simulink model "stablechange"  (R2024b)
settings: Solver=ode45  StartTime=0.0  StopTime=10  FixedStep=1e-5  MaxStep=1e-4  RelTol=1e-3
undefined symbols (not defined in the file): X, Y, Z
libraries: sm_lib x17, nesl_utility x17
settings Model: Creator=lxr  LastModifiedBy=lxr
settings DataIOCC: InspectSignalLogs=on
settings ExplorerConfigSet: InternalSimMechanicsExplorerSettings="<ExplorerConfiguration><canonicalview>default</canonicalview><AnimationSetting><BasePlaybackSpeed>1.0</BasePlaybackSpeed><PlaybackSpeedFactor>1.0</PlaybackSpeedFactor></AnimationSetting><TilePanel><TileInfo><Tiles Columns=\"1\" Count=\"1\" Rows=\"1\"><Column Weight=\"1\"/><Row Weight=\"1\"/><Tile Height=\"1\" Width=\"1\" X=\"0\" Y=\"0\"/></Tiles></TileInfo><SceneInfo><SceneViewer><BGColor><R>0.60000002384185791</R><G>0.60000002384185791</G><B>0.60000002384185791</B></BGColor><Camera><DoPerspective>off</DoPerspective><Position><X>0.439437272864546535</X><Y>-2.25247873719255853</Y><Z>0.67311615033412453</Z></Position><Center><X>0.439437272864546535</X><Y>-2.22044604925031308e-16</Y><Z>0.67311615033412453</Z></Center><Up><X>0</X><Y>-0</Y><Z>1</Z></Up><ViewLimDist>1</ViewLimDist><YLim>3.10627937128803433</YLim><XLim>4.75624821439115486</XLim></Camera></SceneViewer></SceneInfo></TilePanel><MechEditorPanel><Cameras/><GfxPanelCameraMap/><VideoCreator><PlaybackSpeedRatio>1.0</PlaybackSpeedRatio><FrameRate>30</FrameRate><VideoFormat>Motion JPEG AVI</VideoFormat><FrameSize>auto</FrameSize></VideoCreator></MechEditorPanel></ExplorerConfiguration>"

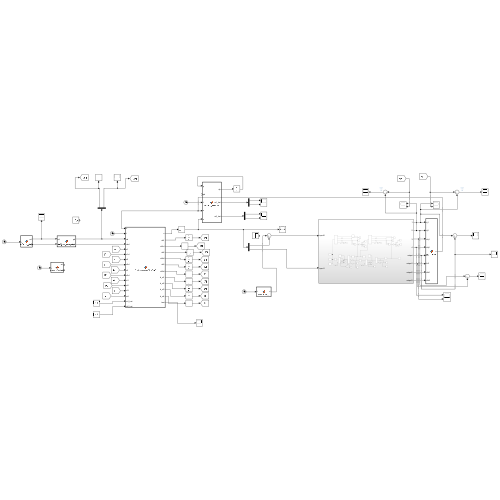
[thumbnail: Simulink's stored preview of the top-level diagram]
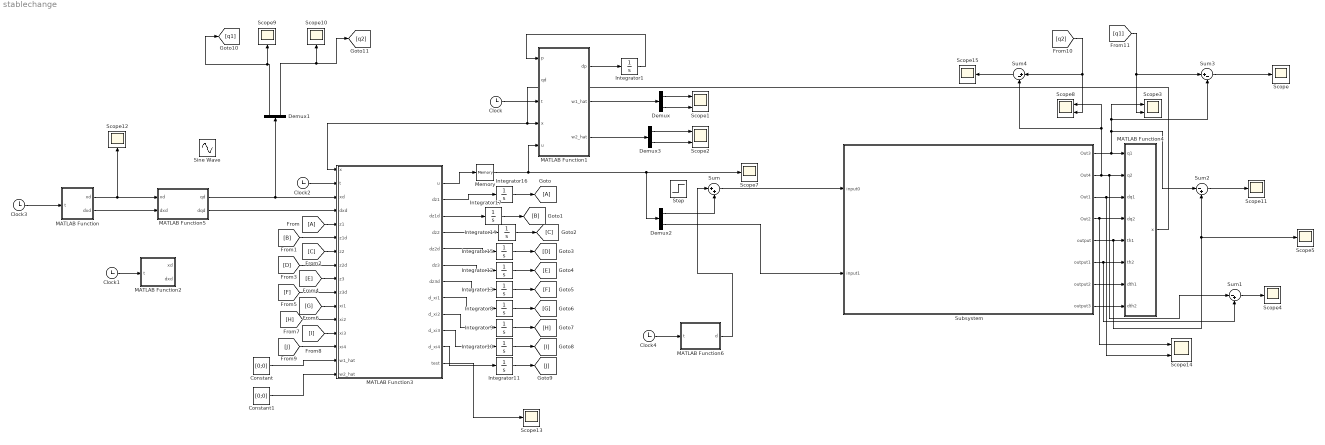
== system stablechange ==
  Clock{,1..4} (5 alike) : Clock
  Constant : Constant  Value=[0;0]
  Constant1 : Constant  Value=[0;0]
  Demux{,1..3} (4 alike) : Demux  Outputs=2
  From : From
  Goto : Goto
  Integrator1 : Integrator  InitialCondition=[0; 0; 0; 0]
  Integrator{8..11,13..17} (9 alike) : Integrator  InitialCondition=[0; 0]
  Integrator12 : Integrator  InitialCondition=[18.5625;135.5175]
  MATLAB Function : MATLAB Function  TreatAsAtomicUnit=on
  MATLAB Function1 : MATLAB Function  TreatAsAtomicUnit=on
  MATLAB Function2 : MATLAB Function  TreatAsAtomicUnit=on
  MATLAB Function3 : MATLAB Function  TreatAsAtomicUnit=on
  MATLAB Function4 : MATLAB Function  TreatAsAtomicUnit=on
  MATLAB Function5 : MATLAB Function  TreatAsAtomicUnit=on
  MATLAB Function6 : MATLAB Function  TreatAsAtomicUnit=on
  Memory : Memory
  Scope{,4..5,7,9..13,15} (10 alike) : Scope
  Scope{1..3,8,14} (5 alike) : Scope  NumInputPorts=2
  Sine Wave : Sin  Amplitude=5  Frequency=100  SampleTime=0
  Step : Step  Time=0  After=5  SampleTime=0
  Subsystem : Subsystem
  Sum : Sum  Inputs=|++
  Sum1 : Sum  Inputs=|-+
  Sum2 : Sum  Inputs=|-+
  Sum3 : Sum  Inputs=|+-
  Sum4 : Sum  Inputs=|+-
  wires:
  MATLAB Function3/11(d_xi4) -> Integrator11/1
  Sum2/1 -> Scope11/1
  MATLAB Function3/9(d_xi2) -> Integrator9/1
  Subsystem/3(Out1) -> Scope14/2, MATLAB Function4/3(dq1)
  [B] -> MATLAB Function3/6(z1d)
  Integrator9/1 -> [H]
  MATLAB Function3/10(d_xi3) -> Integrator10/1
  [J] -> MATLAB Function3/14(xi4)
  Integrator1/1 -> MATLAB Function1/1(p)
  MATLAB Function3/4(dz2) -> Integrator14/1
  Demux1/1 -> [q1], Scope9/1
  Subsystem/8(output3) -> MATLAB Function4/8(dth2)
  Demux2/2 -> Subsystem/2(input1)
  Subsystem/1(Out3) -> Sum2/1, Sum3/2, Scope3/1, MATLAB Function4/1(q1)
  Integrator13/1 -> [F]
  MATLAB Function3/5(dz2d) -> Integrator15/1
  Subsystem/7(output2) -> MATLAB Function4/7(dth1)
  MATLAB Function4/1(x) -> MATLAB Function3/1(x), MATLAB Function1/4(x)
  Integrator15/1 -> [D]
  MATLAB Function3/6(dz3) -> Integrator12/1
  Subsystem/5(output) -> Scope5/1, Sum2/2, MATLAB Function4/5(th1)
  Subsystem/2(Out4) -> Sum4/2, Scope8/1, Sum1/1, MATLAB Function4/2(q2)
  [C] -> MATLAB Function3/7(z2)
  Demux1/2 -> [q2], Scope10/1
  MATLAB Function3/3(dz1d) -> Integrator17/1
  [E] -> MATLAB Function3/9(z3)
  Integrator8/1 -> [G]
  Subsystem/6(output1) -> Sum1/2, MATLAB Function4/6(th2)
  Subsystem/4(Out2) -> Scope14/1, MATLAB Function4/4(dq2)
  From/1 -> MATLAB Function3/5(z1)
  Integrator16/1 -> Goto/1
  MATLAB Function1/1(dp) -> Integrator1/1
  MATLAB Function3/7(dz3d) -> Integrator13/1
  [I] -> MATLAB Function3/13(xi3)
  Integrator10/1 -> [I]
  [H] -> MATLAB Function3/12(xi2)
  Integrator17/1 -> [B]
  MATLAB Function3/2(dz1) -> Integrator16/1
  Integrator11/1 -> [J]
  MATLAB Function3/1(u) -> Memory/1
  Integrator12/1 -> [E]
  MATLAB Function3/8(d_xi1) -> Integrator8/1
  [D] -> MATLAB Function3/8(z2d)
  Integrator14/1 -> [C]
  [G] -> MATLAB Function3/11(xi1)
  [F] -> MATLAB Function3/10(z3d)
  Memory/1 -> MATLAB Function1/5(u), Scope7/1, Demux2/1
  Clock/1 -> MATLAB Function1/3(t)
  MATLAB Function1/2(w1_hat) -> Demux/1
  MATLAB Function1/3(w2_hat) -> Demux3/1
  Clock2/1 -> MATLAB Function3/2(t)
  Demux2/1 -> Sum/2
  Sum/1 -> Subsystem/1(input0)
  [q1] -> Sum3/1, Scope3/2
  [q2] -> Sum4/1, Scope8/2
  Sum1/1 -> Scope4/1
  Clock3/1 -> MATLAB Function/1(t)
  MATLAB Function/1(xd) -> Scope12/1, MATLAB Function5/1(xd)
  MATLAB Function/2(dxd) -> MATLAB Function5/2(dxd)
  MATLAB Function3/12(test) -> Scope13/1
  Sum4/1 -> Scope15/1
  Clock1/1 -> MATLAB Function2/1(t)
  Sum3/1 -> Scope/1
  Clock4/1 -> MATLAB Function6/1(t)
  Demux/1 -> Scope1/1
  Demux/2 -> Scope1/2
  Demux3/1 -> Scope2/1
  Demux3/2 -> Scope2/2
  MATLAB Function5/1(qd) -> Demux1/1, MATLAB Function3/3(xd)
  MATLAB Function5/2(dqd) -> MATLAB Function3/4(dxd)
  MATLAB Function6/1(d) -> Sum/1
  Constant/1 -> MATLAB Function3/15(w1_hat)
  Constant1/1 -> MATLAB Function3/16(w2_hat)

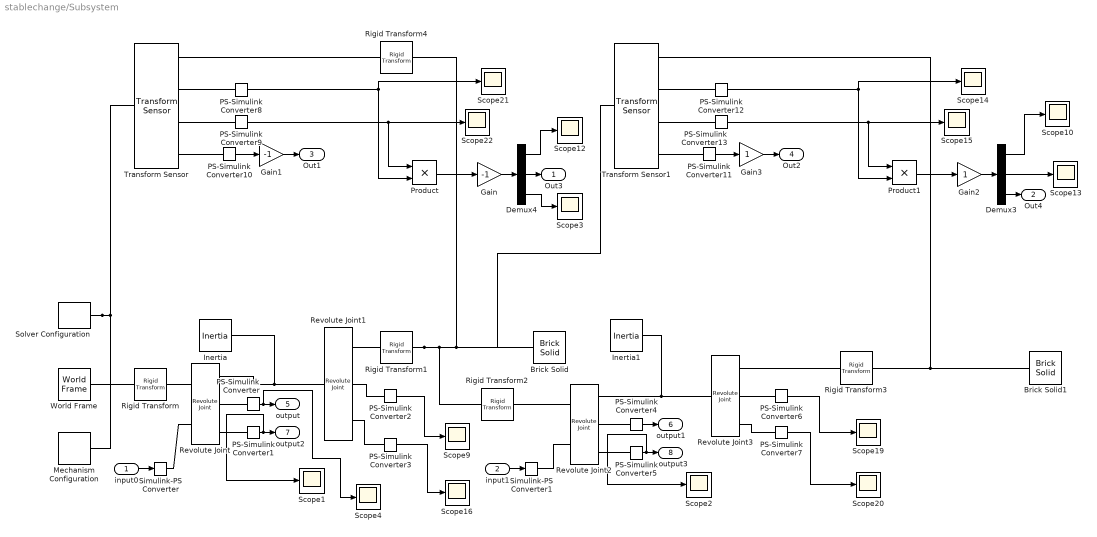
== system stablechange/Subsystem ==
  input0 : Inport
  input1 : Inport  Port=2
  Brick Solid : sm_lib/Body Elements/Brick Solid  BrickDimensions=[0.1 1.05 0.1]  BrickDimensionsUnits=m  ExportEntireGeometry=off  InertiaType=Custom  BasedOnType=Density  Density=1000  DensityUnits=kg/m^3  Mass=2.2  MassUnits=kg  CenterOfMass=[0 0 0]  CenterOfMassUnits=m  MomentsOfInertia=[0 0 0.5]  MomentsOfInertiaUnits=kg*m^2  ProductsOfInertia=[0 0 0]  ProductsOfInertiaUnits=kg*m^2  GraphicType=FromGeometry  MarkerShape=Sphere  MarkerSize=10  GraphicVisPropType=SimpleVisualProperties  GraphicDiffuseColor=[1 1 0]  GraphicOpacity=1.0  GraphicSpecularColor=[0.5 0.5 0.5 1.0]  GraphicAmbientColor=[0.15 0.15 0.15 1.0]  GraphicEmissiveColor=[0.0 0.0 0.0 1.0]  GraphicShininess=75  DoExposeReferenceFrame=on  SerializedFrames=<Frames/>
  Brick Solid1 : sm_lib/Body Elements/Brick Solid  BrickDimensions=[0.1 1.95 0.1]  BrickDimensionsUnits=m  ExportEntireGeometry=off  InertiaType=Custom  BasedOnType=Density  Density=1000  DensityUnits=kg/m^3  Mass=2.8  MassUnits=kg  CenterOfMass=[0 0 0]  CenterOfMassUnits=m  MomentsOfInertia=[0 0 0.5]  MomentsOfInertiaUnits=kg*m^2  ProductsOfInertia=[0 0 0]  ProductsOfInertiaUnits=kg*m^2  GraphicType=FromGeometry  MarkerShape=Sphere  MarkerSize=10  GraphicVisPropType=SimpleVisualProperties  GraphicDiffuseColor=[1 0 0]  GraphicOpacity=1.0  GraphicSpecularColor=[0.5 0.5 0.5 1.0]  GraphicAmbientColor=[0.15 0.15 0.15 1.0]  GraphicEmissiveColor=[0.0 0.0 0.0 1.0]  GraphicShininess=75  DoExposeReferenceFrame=on  SerializedFrames=<Frames/>
  Demux3 : Demux  Outputs=3
  Demux4 : Demux  Outputs=3
  Gain : Gain  Gain=-1
  Gain1 : Gain  Gain=-1
  Gain2 : Gain
  Gain3 : Gain
  Inertia : sm_lib/Body Elements/Inertia  InertiaType=Custom  Mass=0  MassUnits=kg  CenterOfMass=[0 0 0]  CenterOfMassUnits=m  MomentsOfInertia=[0 0 0.005]  MomentsOfInertiaUnits=kg*m^2  ProductsOfInertia=[0 0 0]  ProductsOfInertiaUnits=kg*m^2  GraphicType=Marker  MarkerShape=Inertia  MarkerSize=20  GraphicVisPropType=SimpleVisualProperties  GraphicDiffuseColor=[0.5 0.5 0.5]  GraphicOpacity=1  GraphicSpecularColor=[0.5 0.5 0.5 1.0]  GraphicAmbientColor=[0.15 0.15 0.15 1.0]  GraphicEmissiveColor=[0.0 0.0 0.0 1.0]  GraphicShininess=75
  Inertia1 : sm_lib/Body Elements/Inertia  InertiaType=Custom  Mass=0  MassUnits=kg  CenterOfMass=[0 0 0]  CenterOfMassUnits=m  MomentsOfInertia=[0 0 0.005]  MomentsOfInertiaUnits=kg*m^2  ProductsOfInertia=[0 0 0]  ProductsOfInertiaUnits=kg*m^2  GraphicType=Marker  MarkerShape=Inertia  MarkerSize=20  GraphicVisPropType=SimpleVisualProperties  GraphicDiffuseColor=[0.5 0.5 0.5]  GraphicOpacity=1  GraphicSpecularColor=[0.5 0.5 0.5 1.0]  GraphicAmbientColor=[0.15 0.15 0.15 1.0]  GraphicEmissiveColor=[0.0 0.0 0.0 1.0]  GraphicShininess=75
  Mechanism Configuration : sm_lib/Utilities/Mechanism Configuration  UniformGravity=Constant  GravityVector=[0 0 -9.81]  GravityVectorUnits=m/s^2  LinearizationDelta=0.001  JointModeTransitionNonlinearIterations=2
  PS-Simulink Converter{,1..13} (14 alike) : nesl_utility/PS-Simulink Converter  PhysicalDomain=network_engine_domain  SubClassName=ps_output  LeftPortType=input  RightPortType=output  PseudoPeriodic=off  Frequencies=[]  VectorFormat=inherit  Unit=inherit  AffineConversion=off
  Product : Product
  Product1 : Product
  Revolute Joint : sm_lib/Joints/Revolute Joint  JointMode=Normal  CompositeWrenchDir=FollowerOnBase  CompositeWrenchFrame=BaseFrame  SenseConstraintForce=off  SenseConstraintTorque=off  SenseTotalForce=off  SenseTotalTorque=off  PositionTargetSpecify=off  PositionTargetPriority=High  PositionTargetValue=0  PositionTargetValueUnits=deg  VelocityTargetSpecify=off  VelocityTargetPriority=High  VelocityTargetValue=0  VelocityTargetValueUnits=deg/s  EquilibriumPosition=0  EquilibriumPositionUnits=deg  SpringStiffness=0  SpringStiffnessUnits=N*m/deg  DampingCoefficient=0  DampingCoefficientUnits=N*m*s/rad  LowerLimitSpecify=off  LowerLimitBound=-90  LowerLimitBoundUnits=deg  LowerLimitStiffness=1e4  LowerLimitStiffnessUnits=N*m/deg  LowerLimitDamping=10  LowerLimitDampingUnits=N*m/(deg/s)  LowerLimitTransitionRegionWidth=0.1  LowerLimitTransitionRegionWidthUnits=deg  UpperLimitSpecify=off  UpperLimitBound=90  UpperLimitBoundUnits=deg  UpperLimitStiffness=1e4  UpperLimitStiffnessUnits=N*m/deg  UpperLimitDamping=10  UpperLimitDampingUnits=N*m/(deg/s)  UpperLimitTransitionRegionWidth=0.1  UpperLimitTransitionRegionWidthUnits=deg  TorqueActuationMode=InputTorque  MotionActuationMode=ComputedMotion  SensePosition=on  SenseVelocity=on  SenseAcceleration=off  SenseTorqueForce=off  SenseLowerLimitTorqueForce=off  SenseUpperLimitTorqueForce=off
  Revolute Joint1 : sm_lib/Joints/Revolute Joint  JointMode=Normal  CompositeWrenchDir=FollowerOnBase  CompositeWrenchFrame=BaseFrame  SenseConstraintForce=off  SenseConstraintTorque=off  SenseTotalForce=off  SenseTotalTorque=off  PositionTargetSpecify=on  PositionTargetPriority=High  PositionTargetValue=0  PositionTargetValueUnits=deg  VelocityTargetSpecify=off  VelocityTargetPriority=High  VelocityTargetValue=0  VelocityTargetValueUnits=deg/s  EquilibriumPosition=0  EquilibriumPositionUnits=deg  SpringStiffness=100  SpringStiffnessUnits=N*m/rad  DampingCoefficient=1  DampingCoefficientUnits=N*m*s/rad  LowerLimitSpecify=off  LowerLimitBound=-90  LowerLimitBoundUnits=deg  LowerLimitStiffness=1e4  LowerLimitStiffnessUnits=N*m/deg  LowerLimitDamping=10  LowerLimitDampingUnits=N*m/(deg/s)  LowerLimitTransitionRegionWidth=0.1  LowerLimitTransitionRegionWidthUnits=deg  UpperLimitSpecify=off  UpperLimitBound=90  UpperLimitBoundUnits=deg  UpperLimitStiffness=1e4  UpperLimitStiffnessUnits=N*m/deg  UpperLimitDamping=10  UpperLimitDampingUnits=N*m/(deg/s)  UpperLimitTransitionRegionWidth=0.1  UpperLimitTransitionRegionWidthUnits=deg  TorqueActuationMode=NoTorque  MotionActuationMode=ComputedMotion  SensePosition=on  SenseVelocity=on  SenseAcceleration=off  SenseTorqueForce=off  SenseLowerLimitTorqueForce=off  SenseUpperLimitTorqueForce=off
  Revolute Joint2 : sm_lib/Joints/Revolute Joint  JointMode=Normal  CompositeWrenchDir=FollowerOnBase  CompositeWrenchFrame=BaseFrame  SenseConstraintForce=off  SenseConstraintTorque=off  SenseTotalForce=off  SenseTotalTorque=off  PositionTargetSpecify=off  PositionTargetPriority=High  PositionTargetValue=0  PositionTargetValueUnits=deg  VelocityTargetSpecify=off  VelocityTargetPriority=High  VelocityTargetValue=0  VelocityTargetValueUnits=deg/s  EquilibriumPosition=0  EquilibriumPositionUnits=deg  SpringStiffness=0  SpringStiffnessUnits=N*m/deg  DampingCoefficient=0  DampingCoefficientUnits=N*m*s/rad  LowerLimitSpecify=off  LowerLimitBound=-90  LowerLimitBoundUnits=deg  LowerLimitStiffness=1e4  LowerLimitStiffnessUnits=N*m/deg  LowerLimitDamping=10  LowerLimitDampingUnits=N*m/(deg/s)  LowerLimitTransitionRegionWidth=0.1  LowerLimitTransitionRegionWidthUnits=deg  UpperLimitSpecify=off  UpperLimitBound=90  UpperLimitBoundUnits=deg  UpperLimitStiffness=1e4  UpperLimitStiffnessUnits=N*m/deg  UpperLimitDamping=10  UpperLimitDampingUnits=N*m/(deg/s)  UpperLimitTransitionRegionWidth=0.1  UpperLimitTransitionRegionWidthUnits=deg  TorqueActuationMode=InputTorque  MotionActuationMode=ComputedMotion  SensePosition=on  SenseVelocity=on  SenseAcceleration=off  SenseTorqueForce=off  SenseLowerLimitTorqueForce=off  SenseUpperLimitTorqueForce=off
  Revolute Joint3 : sm_lib/Joints/Revolute Joint  JointMode=Normal  CompositeWrenchDir=FollowerOnBase  CompositeWrenchFrame=BaseFrame  SenseConstraintForce=off  SenseConstraintTorque=off  SenseTotalForce=off  SenseTotalTorque=off  PositionTargetSpecify=off  PositionTargetPriority=High  PositionTargetValue=0  PositionTargetValueUnits=deg  VelocityTargetSpecify=off  VelocityTargetPriority=High  VelocityTargetValue=0  VelocityTargetValueUnits=deg/s  EquilibriumPosition=0  EquilibriumPositionUnits=deg  SpringStiffness=100  SpringStiffnessUnits=N*m/rad  DampingCoefficient=1  DampingCoefficientUnits=N*m*s/rad  LowerLimitSpecify=off  LowerLimitBound=-90  LowerLimitBoundUnits=deg  LowerLimitStiffness=1e4  LowerLimitStiffnessUnits=N*m/deg  LowerLimitDamping=10  LowerLimitDampingUnits=N*m/(deg/s)  LowerLimitTransitionRegionWidth=0.1  LowerLimitTransitionRegionWidthUnits=deg  UpperLimitSpecify=off  UpperLimitBound=90  UpperLimitBoundUnits=deg  UpperLimitStiffness=1e4  UpperLimitStiffnessUnits=N*m/deg  UpperLimitDamping=10  UpperLimitDampingUnits=N*m/(deg/s)  UpperLimitTransitionRegionWidth=0.1  UpperLimitTransitionRegionWidthUnits=deg  TorqueActuationMode=NoTorque  MotionActuationMode=ComputedMotion  SensePosition=on  SenseVelocity=on  SenseAcceleration=off  SenseTorqueForce=off  SenseLowerLimitTorqueForce=off  SenseUpperLimitTorqueForce=off
  Rigid Transform : sm_lib/Frames and Transforms/Rigid Transform  RotationMethod=StandardAxis  FollAlignAxisA=+X  BaseAlignAxisA=+Y  FollAlignAxisB=+Y  BaseAlignAxisB=+Z  RotationStandardAxis=+X  RotationAngle=90  RotationAngleUnits=deg  RotationArbitraryAxis=[0 0 1]  RotationSequenceAxes=FollowerAxes  RotationSequence=XYX  RotationSequenceAngles=[0 0 0]  RotationSequenceAnglesUnits=deg  RotationMatrix=[1 0 0; 0 1 0; 0 0 1]  Quaternion=[1 0 0 0]  TranslationMethod=None  TranslationCartesianOffset=[0 0 0]  TranslationCartesianOffsetUnits=m  TranslationStandardAxis=+Z  TranslationStandardOffset=0  TranslationStandardOffsetUnits=m  TranslationROffset=0  TranslationROffsetUnits=m  TranslationThetaOffset=0  TranslationThetaOffsetUnits=deg  TranslationZOffset=0  TranslationZOffsetUnits=m
  Rigid Transform1 : sm_lib/Frames and Transforms/Rigid Transform  RotationMethod=None  FollAlignAxisA=+X  BaseAlignAxisA=+Y  FollAlignAxisB=+Y  BaseAlignAxisB=+Z  RotationStandardAxis=+X  RotationAngle=90  RotationAngleUnits=deg  RotationArbitraryAxis=[0 0 1]  RotationSequenceAxes=FollowerAxes  RotationSequence=XYX  RotationSequenceAngles=[0 0 0]  RotationSequenceAnglesUnits=deg  RotationMatrix=[1 0 0; 0 1 0; 0 0 1]  Quaternion=[1 0 0 0]  TranslationMethod=StandardAxis  TranslationCartesianOffset=[0 0 0]  TranslationCartesianOffsetUnits=m  TranslationStandardAxis=-Y  TranslationStandardOffset=0.5  TranslationStandardOffsetUnits=m  TranslationROffset=0  TranslationROffsetUnits=m  TranslationThetaOffset=0  TranslationThetaOffsetUnits=deg  TranslationZOffset=0  TranslationZOffsetUnits=m
  Rigid Transform2 : sm_lib/Frames and Transforms/Rigid Transform  RotationMethod=None  FollAlignAxisA=+X  BaseAlignAxisA=+Y  FollAlignAxisB=+Y  BaseAlignAxisB=+Z  RotationStandardAxis=+X  RotationAngle=90  RotationAngleUnits=deg  RotationArbitraryAxis=[0 0 1]  RotationSequenceAxes=FollowerAxes  RotationSequence=XYX  RotationSequenceAngles=[0 0 0]  RotationSequenceAnglesUnits=deg  RotationMatrix=[1 0 0; 0 1 0; 0 0 1]  Quaternion=[1 0 0 0]  TranslationMethod=StandardAxis  TranslationCartesianOffset=[0 0 0]  TranslationCartesianOffsetUnits=m  TranslationStandardAxis=-Y  TranslationStandardOffset=0.5  TranslationStandardOffsetUnits=m  TranslationROffset=0  TranslationROffsetUnits=m  TranslationThetaOffset=0  TranslationThetaOffsetUnits=deg  TranslationZOffset=0  TranslationZOffsetUnits=m
  Rigid Transform3 : sm_lib/Frames and Transforms/Rigid Transform  RotationMethod=None  FollAlignAxisA=+X  BaseAlignAxisA=+Y  FollAlignAxisB=+Y  BaseAlignAxisB=+Z  RotationStandardAxis=+X  RotationAngle=90  RotationAngleUnits=deg  RotationArbitraryAxis=[0 0 1]  RotationSequenceAxes=FollowerAxes  RotationSequence=XYX  RotationSequenceAngles=[0 0 0]  RotationSequenceAnglesUnits=deg  RotationMatrix=[1 0 0; 0 1 0; 0 0 1]  Quaternion=[1 0 0 0]  TranslationMethod=StandardAxis  TranslationCartesianOffset=[0 0 0]  TranslationCartesianOffsetUnits=m  TranslationStandardAxis=-Y  TranslationStandardOffset=1  TranslationStandardOffsetUnits=m  TranslationROffset=0  TranslationROffsetUnits=m  TranslationThetaOffset=0  TranslationThetaOffsetUnits=deg  TranslationZOffset=0  TranslationZOffsetUnits=m
  Rigid Transform4 : sm_lib/Frames and Transforms/Rigid Transform  RotationMethod=StandardAxis  FollAlignAxisA=+X  BaseAlignAxisA=+Y  FollAlignAxisB=+Y  BaseAlignAxisB=+Z  RotationStandardAxis=-X  RotationAngle=90  RotationAngleUnits=deg  RotationArbitraryAxis=[0 0 1]  RotationSequenceAxes=FollowerAxes  RotationSequence=XYX  RotationSequenceAngles=[0 0 0]  RotationSequenceAnglesUnits=deg  RotationMatrix=[1 0 0; 0 1 0; 0 0 1]  Quaternion=[1 0 0 0]  TranslationMethod=None  TranslationCartesianOffset=[0 0 0]  TranslationCartesianOffsetUnits=m  TranslationStandardAxis=+Z  TranslationStandardOffset=0  TranslationStandardOffsetUnits=m  TranslationROffset=0  TranslationROffsetUnits=m  TranslationThetaOffset=0  TranslationThetaOffsetUnits=deg  TranslationZOffset=0  TranslationZOffsetUnits=m
  Scope{1..4,9..10,12..16,19..22} (15 alike) : Scope
  Simulink-PS Converter : nesl_utility/Simulink-PS Converter  PhysicalDomain=network_engine_domain  SubClassName=ps_input  LeftPortType=input  RightPortType=output  PseudoPeriodic=off  Frequencies=[]  NoiseDistribution=none  NoiseParameters=[]  Unit=1  AffineConversion=off  FilteringAndDerivatives=provide  SimscapeFilterOrder=1  InputFilterTimeConstant=0.001  UdotUserProvided=0
  Simulink-PS Converter1 : nesl_utility/Simulink-PS Converter  PhysicalDomain=network_engine_domain  SubClassName=ps_input  LeftPortType=input  RightPortType=output  PseudoPeriodic=off  Frequencies=[]  NoiseDistribution=none  NoiseParameters=[]  Unit=1  AffineConversion=off  FilteringAndDerivatives=provide  SimscapeFilterOrder=1  InputFilterTimeConstant=0.001  UdotUserProvided=0
  Solver Configuration : nesl_utility/Solver Configuration  PhysicalDomain=network_engine_domain  SubClassName=solver  LeftPortType=input  RightPortType=generic  Tones=[]  Harmonics=[]  SimulateNoise=off  Profile=off  UseLocalSampling=off  EnableSwitchedLinearOptims=on  FrequencyDomain=off  UseCCode=off  RelTol=0.001  AbsTol=1e-06  MinStep=1e-09  ToWorkspace=off  RevertToSquareIcSolve=off  NumHomotopyIterations=100  PhasorMode=off  PhasorModeNumHarmonics=1  ConsistencySolver=NEWTON_XTOL_AFTER_FTOL  IndexReductionMethod=DerivativeReplacement  DoDC=off  ResidualTolerance=1e-09  ConsistencyTolSource=GLOBAL  ConsistencyAbsTol=0.001  ConsistencyRelTol=0.001  ConsistencyTolFactor=0.001  UseLocalSolver=off  LocalSolverChoice=NE_BACKWARD_EULER_ADVANCER  ResolveIndetEquations=on  FunctionEvalNumThread=1  LocalSolverSampleTime=0.001  DoFixedCost=off  MaxNonlinIter=3  MaxModeIter=2  ComputeImpulses=off  ImpulseIterations=2  LinearAlgebra=Sparse  LinearAlgebraNumThread=0  EquationFormulation=NE_TIME_EF  DelaysMemoryBudget=1024  AutomaticFiltering=on  FilteringTimeConstant=0.001  PartitionStorageMethod=AS_NEEDED  PartitionMemoryBudget=1024  PartitionMethod=FAST  MultibodyUseLocalSolver=off  MultibodyLocalSolverChoice=ODE1  MultibodyLocalSolverSampleTime=0.001
  Transform Sensor : sm_lib/Frames and Transforms/Transform Sensor  MeasurementFrame=World  RotationSequence=ZXY  SenseAngle=on  SenseAxis=on  SenseQ=off  SenseR=off  SenseRotationSequence=off  SenseOmegaX=off  SenseOmegaY=on  SenseOmegaZ=off  SenseOmega=off  SenseQDot=off  SenseRDot=off  SenseRotationSequenceDot=off  SenseAlphaX=off  SenseAlphaY=off  SenseAlphaZ=off  SenseAlpha=off  SenseQDDot=off  SenseRDDot=off  SenseX=off  SenseY=off  SenseZ=off  SenseXYZ=off  SenseRad=off  SenseAzim=off  SenseDist=off  SenseInc=off  SenseXDot=off  SenseYDot=off  SenseZDot=off  SenseXYZDot=off  SenseRadDot=off  SenseAzimDot=off  SenseDistDot=off  SenseIncDot=off  SenseXDDot=off  SenseYDDot=off  SenseZDDot=off  SenseXYZDDot=off  SenseRadDDot=off  SenseAzimDDot=off  SenseDistDDot=off  SenseIncDDot=off
  Transform Sensor1 : sm_lib/Frames and Transforms/Transform Sensor  MeasurementFrame=Follower  RotationSequence=ZXY  SenseAngle=on  SenseAxis=on  SenseQ=off  SenseR=off  SenseRotationSequence=off  SenseOmegaX=off  SenseOmegaY=off  SenseOmegaZ=on  SenseOmega=off  SenseQDot=off  SenseRDot=off  SenseRotationSequenceDot=off  SenseAlphaX=off  SenseAlphaY=off  SenseAlphaZ=off  SenseAlpha=off  SenseQDDot=off  SenseRDDot=off  SenseX=off  SenseY=off  SenseZ=off  SenseXYZ=off  SenseRad=off  SenseAzim=off  SenseDist=off  SenseInc=off  SenseXDot=off  SenseYDot=off  SenseZDot=off  SenseXYZDot=off  SenseRadDot=off  SenseAzimDot=off  SenseDistDot=off  SenseIncDot=off  SenseXDDot=off  SenseYDDot=off  SenseZDDot=off  SenseXYZDDot=off  SenseRadDDot=off  SenseAzimDDot=off  SenseDistDDot=off  SenseIncDDot=off
  World Frame : sm_lib/Frames and Transforms/World Frame
  Out3 : Outport
  Out4 : Outport  Port=2
  Out1 : Outport  Port=3
  Out2 : Outport  Port=4
  output : Outport  Port=5
  output1 : Outport  Port=6
  output2 : Outport  Port=7
  output3 : Outport  Port=8
  wires:
  input1/1 -> Simulink-PS Converter1/1
  PS-Simulink Converter12/1 -> Scope14/1, Product1/2
  PS-Simulink Converter13/1 -> Product1/1, Scope15/1
  PS-Simulink Converter3/1 -> Scope16/1
  Gain1/1 -> Out1/1
  Gain2/1 -> Demux3/1
  PS-Simulink Converter8/1 -> Scope21/1, Product/2
  Demux4/3 -> Scope3/1
  Demux3/1 -> Scope10/1
  PS-Simulink Converter9/1 -> Product/1, Scope22/1
  Product1/1 -> Gain2/1
  Gain/1 -> Demux4/1
  PS-Simulink Converter4/1 -> output1/1
  PS-Simulink Converter7/1 -> Scope20/1
  PS-Simulink Converter1/1 -> Scope1/1, output2/1
  PS-Simulink Converter2/1 -> Scope9/1
  PS-Simulink Converter11/1 -> Gain3/1
  PS-Simulink Converter10/1 -> Gain1/1
  Demux3/3 -> Out4/1
  Product/1 -> Gain/1
  PS-Simulink Converter6/1 -> Scope19/1
  Demux4/1 -> Scope12/1
  PS-Simulink Converter5/1 -> Scope2/1, output3/1
  Demux3/2 -> Scope13/1
  PS-Simulink Converter/1 -> Scope4/1, output/1
  Gain3/1 -> Out2/1
  input0/1 -> Simulink-PS Converter/1
  Demux4/2 -> Out3/1
  connections:
  Revolute Joint2/LConn1 -- Rigid Transform2/RConn1
  Revolute Joint3/LConn1 -- Inertia1/RConn1 -- Revolute Joint2/RConn1
  Solver Configuration/RConn1 -- Transform Sensor/LConn1 -- Rigid Transform/LConn1 -- Mechanism Configuration/RConn1 -- World Frame/RConn1
  Revolute Joint/LConn1 -- Rigid Transform/RConn1
  PS-Simulink Converter2/LConn1 -- Revolute Joint1/RConn2
  Rigid Transform1/RConn1 -- Rigid Transform2/LConn1 -- Transform Sensor1/LConn1 -- Brick Solid/RConn1 -- Rigid Transform4/LConn1
  Transform Sensor/RConn4 -- PS-Simulink Converter10/LConn1
  PS-Simulink Converter13/LConn1 -- Transform Sensor1/RConn3
  Revolute Joint1/LConn1 -- Inertia/RConn1 -- Revolute Joint/RConn1
  PS-Simulink Converter7/LConn1 -- Revolute Joint3/RConn3
  Revolute Joint/LConn2 -- Simulink-PS Converter/RConn1
  PS-Simulink Converter12/LConn1 -- Transform Sensor1/RConn2
  Simulink-PS Converter1/RConn1 -- Revolute Joint2/LConn2
  PS-Simulink Converter4/LConn1 -- Revolute Joint2/RConn2
  PS-Simulink Converter5/LConn1 -- Revolute Joint2/RConn3
  Rigid Transform4/RConn1 -- Transform Sensor/RConn1
  PS-Simulink Converter6/LConn1 -- Revolute Joint3/RConn2
  PS-Simulink Converter9/LConn1 -- Transform Sensor/RConn3
  Brick Solid1/RConn1 -- Transform Sensor1/RConn1 -- Rigid Transform3/RConn1
  PS-Simulink Converter1/LConn1 -- Revolute Joint/RConn3
  Revolute Joint1/RConn3 -- PS-Simulink Converter3/LConn1
  PS-Simulink Converter/LConn1 -- Revolute Joint/RConn2
  PS-Simulink Converter8/LConn1 -- Transform Sensor/RConn2
  Rigid Transform3/LConn1 -- Revolute Joint3/RConn1
  Rigid Transform1/LConn1 -- Revolute Joint1/RConn1
  Transform Sensor1/RConn4 -- PS-Simulink Converter11/LConn1

== matlab function stablechange/MATLAB Function5 ==
  settings: updateMethod=DISCRETE
  data: xd input; qd output; dqd output; dxd input
function [qd, dqd] = ee2joint_onepoint(xd, dxd)
% Input:
%   xd   - [2×1] current end-effector position [x; z]
%   dxd  - [2×1] current end-effector velocity [dx; dz]
% Output:
%   qd   - [2×1] current joint angles [q1; q2]
%   dqd  - [2×1] current joint velocities [dq1; dq2]

    % Manipulator parameters
    l1 = 1.05;
    l2 = 1.95;

    x = xd(1);
    z = xd(2);

    % --------- Inverse kinematics (using fixed elbow-down solution) ---------
    r2 = x^2 + z^2;
    cos_q2 = (r2 - l1^2 - l2^2) / (2 * l1 * l2);
    cos_q2 = min(max(cos_q2, -1), 1);  % constrain within [-1, 1]

    q2 = acos(cos_q2);  % fixed elbow-down solution
    k1 = l1 + l2 * cos(q2);
    k2 = l2 * sin(q2);
    q1 = atan2(z, x) - atan2(k2, k1);

    qd = [q1; q2];

    % --------- Jacobian for joint velocities ---------
    J = [ ...
        -l1*sin(q1) - l2*sin(q1 + q2),  -l2*sin(q1 + q2);
         l1*cos(q1) + l2*cos(q1 + q2),   l2*cos(q1 + q2) ];

    dqd = pinv(J) * dxd;

end

== matlab function stablechange/MATLAB Function6 ==
  data: t input; d output
function d = disturbance(t)

% Initialization
d = 0;

% ==== Disturbance segment example ====
% Add high-frequency disturbance between 2s and 4s
if t >= 2 && t <= 4
    d = 10 * sin(100 * t);  % High-frequency disturbance, frequency 100 Hz, amplitude 3
end

% ==== Step disturbance example ====
% Add a sudden disturbance at 6s
if t >= 5 && t <= 6
    d = d + 5;  % Add a sudden or step disturbance
end

% ==== Frequency sweep disturbance example ====
% From 7s to 9s, use a disturbance with varying frequency (chirp-like)
if t >= 7 && t <= 9
    d = d + 5 * sin(30 * t^2);  % Frequency increases with t^2
end

end

== matlab function stablechange/MATLAB Function1 ==
  data: p input; qd input; t input; x input; u input size=[2,1]; dp output; w1_hat output; w2_hat output
function [dp, w1_hat, w2_hat] = RESO_module(p,qd,t, x, u)
% === RESO module ===
% Input:
%   p : state variables [p1; p2] ∈ ℝ⁴
%   x : actual system states [q1; q2; dq1; dq2; th1; th2; dth1; dth2] ∈ ℝ⁸
%   u : control input [u1; u2] ∈ ℝ²
% Output:
%   dz      : derivative of z [dp1; dp2] ∈ ℝ⁴
%   w1_hat  : estimated disturbance 1 ∈ ℝ²
%   w2_hat  : estimated disturbance 2 ∈ ℝ²

% ========== Nominal controller parameters (from paper) ==========
 % --- Parameters ---
    % m1 = 2;  m2 = 3;
    % L1 = 1;  L2 = 2;
    % Lc1 = 0.5; Lc2 = 1;
    % I1 = 0.5;    I2 = 0.5;
% g  = 9.81;

K0 = diag([100, 100]);
J0 = diag([0.005, 0.005]);

% ========== Input decomposition ==========
% ========================
% Unpack state variables
% ========================
q1 = x(1);
q2 = x(2);
q1_dot = x(3);
q2_dot = x(4);
theta1 = x(5);
theta2 = x(6);
theta1_dot = x(7);
theta2_dot = x(8);

% State variable organization
q  = [q1; q2];                        %x1
dq = [q1_dot; q2_dot];                %x2
theta = [theta1; theta2];             %x3
dtheta = [theta1_dot; theta2_dot];    %x4
% p11 = p(1); p12 = p(2);
% p21 = p(3); p22 = p(4);
% p1 = [p11;p12];
% p2 = [p21;p22];
p1 = p(1:2);
p2 = p(3:4);

m1 = 2.2; m2 = 2.8; l1 = 1.05; l2 = 1.95; g = 9.81;lc1=l1/2;lc2=l2/2;
I1 = 0.5; I2 = 0.5;

a1 = m1*lc1^2 + m2*l1^2 + I1;
a2 = m2*lc2^2 + I2;
a3 = m2*l1*lc2;
a4 = (m1*lc1 + m2*l1)*g;
a5 = m2*g*lc2;
% a1 = 4.0;
% a2 = 3.5;
% a3 = 3.0;
% a4 = 39.24;
% a5 = 29.43;
% ------------------------
% Mass matrix M(q)
% ------------------------
M11 = a1 + a2 + 2 * a3 * cos(q2);
M12 = a2 + a3 * cos(q2);
M21 = M12;
M22 = a2;

M0 = [M11, M12;
     M21, M22];

% ------------------------
% Coriolis/centrifugal matrix C(q, dq)
% ------------------------
C11 = -a3 * q2_dot * sin(q2);
C12 = -a3 * (q1_dot + q2_dot) * sin(q2);
C21 =  a3 * q1_dot * sin(q2);
C22 = 0;

C0 = [C11, C12;
     C21, C22];

% ------------------------
% Gravity term G(q)
% ------------------------
G1 = a4 * sin(q1) + a5 * sin(q1 + q2);
G2 = a5 * sin(q1 + q2);
G0 = [G1;
     G2];

% Observer gains (diagonal constants in the paper)
% beta1 = 80;                     % tunable parameter
% beta2 = 80;

beta_max = 80;
% c = 2;                % growth rate (larger → faster convergence)
% beta1 = beta_max * (1 - exp(-c * t));
lambda = 0.3;       % warm start speed
gamma = 0.05;      % adaptive response strength
e0 = 0.1;         % avoid division by zero, normalization
% Error calculation
e_q = norm(q - qd);  % tracking error
% Warm start term
warm_start = 1 - exp(-lambda * t);
% Adaptive adjustment term
adapt_term = 1 + gamma * (e_q / (e0 + e_q));
% Combined
beta1 = beta_max * warm_start * adapt_term;

lambda2 = 0.3;       % warm start speed
gamma2 = 0.05;      % adaptive response strength

% Warm start term
warm_start2 = 1 - exp(-lambda2 * t);
% Adaptive adjustment term
adapt_term2 = 1 + gamma2 * (e_q / (e0 + e_q));
% Combined
beta2 = beta_max * warm_start2 * adapt_term2;

% ========== f1, f2 according to equation (12) in the paper ==========
f1 = -M0 \ (C0 * dq + G0 + K0 * q);
% f1 = -M0 \ (C0 * dq + K0 * q);
f2 = J0 \ K0 * (q - theta);

% ========== RESO differential equations (equation 13 in the paper) ==========
dp1 = -beta1 * p1 - beta1^2 * dq - beta1 * (M0 \ K0 * theta + f1);
dp2 = -beta2 * p2 - beta2^2 * dtheta - beta2 * (J0 \ u + f2);

% ========== Disturbance estimation output ==========
w1_hat = p1 + beta1 * dq;
w2_hat = p2 + beta2 * dtheta;

% ========== Pack output ==========
dp = [dp1;
      dp2];
end

== matlab function stablechange/MATLAB Function ==
  data: t input; xd output; dxd output
function [xd, dxd] = end_effector_trajectory(t)
% Trajectory generator: input joint angles (in degrees), output smooth end-effector trajectory [x; z]
%
% Input:
%   t            - current time
%   q_start_deg  - initial joint angles [q1_deg; q2_deg]
%   q_goal_deg   - target joint angles [q1_deg; q2_deg]
%
% Output:
%   xd  - current end-effector position [x; z]
%   dxd - current end-effector velocity [dx; dz]
q_start_deg = [0; 0];
q_goal_deg  = [30; 60];

    % Manipulator parameters
    l1 = 1.05;
    l2 = 1.95;

    % Total time
    T = 8;

    % Constrain time range
    t = max(0, min(t, T));
    tau = t / T;

    % Convert angles to radians
    q_start = deg2rad(q_start_deg);
    q_goal  = deg2rad(q_goal_deg);

    % --- Forward kinematics function ---
    fk = @(q) [ ...
        l1 * cos(q(1)) + l2 * cos(q(1) + q(2));
        l1 * sin(q(1)) + l2 * sin(q(1) + q(2)) ];

    % --- Initial and target end-effector positions ---
    p0 = fk(q_start);
    pf = fk(q_goal);

    % Quintic polynomial S-curve interpolation
    s  = 10*tau^3 - 15*tau^4 + 6*tau^5;
    ds = (30*tau^2 - 60*tau^3 + 30*tau^4) / T;

    % Interpolated position and velocity
    xd  = p0 + (pf - p0) * s;
    dxd = (pf - p0) * ds;

end

== matlab function stablechange/MATLAB Function2 ==
  data: t input; xd output; dxd output
function [xd, dxd] = ReferenceGenerator(t)

% === Reference trajectory (main trajectory) ===
xd1 = sin(t);
xd2 = 0.6 * (sin(t) + sin(2*t));

% === Add small-amplitude high-frequency disturbances ===
xd1 = xd1 + 0.05 * sin(100*t);     % approx. 3.2 Hz
xd2 = xd2 + 0.05 * sin(25*t);      % approx. 4 Hz

xd = [xd1; xd2];

% === First derivative (velocity) ===
dxd1 = cos(t) + 0.05 * 100 * cos(100*t);
dxd2 = 0.6 * (cos(t) + 2*cos(2*t)) + 0.05 * 25 * cos(25*t);

dxd = [dxd1; dxd2];

end

== matlab function stablechange/MATLAB Function3 ==
  data: x input; t input; xd input; dxd input; z1 input; z1d input; z2 input; z2d input; z3 input; z3d input; xi1 input; xi2 input; xi3 input; xi4 input; u output; dz1 output; dz1d output; dz2 output; dz2d output; dz3 output; dz3d output; w1_hat input; w2_hat input; d_xi1 output; d_xi2 output; d_xi3 output; d_xi4 output; test output
function [u, dz1, dz1d, dz2, dz2d, dz3, dz3d, d_xi1, d_xi2, d_xi3, d_xi4, test] = BacksteppingWithSCF( ...
    x, t,xd, dxd, ...
    z1, z1d, z2, z2d, z3, z3d, ...
    xi1, xi2, xi3, xi4, ...
    w1_hat, w2_hat)

% ==== Parameters ====
% Control gains
k1 = diag([30, 30]);
k2 = diag([30, 30]);
k3 = diag([30, 30]);
k4 = diag([15, 15]);

% Filter parameters
zeta = diag([0.8, 0.8]);
omega_n = diag([1500, 1500]);

% Manipulator parameters (control model)
K0 = diag([100, 100]);
J0 = diag([0.005, 0.005]);

m1 = 2.2; m2 = 2.8; l1 = 1.05; l2 = 1.95; g = 9.81;lc1=l1/2;lc2=l2/2;
I1 = 0.5; I2 = 0.5;

% ==== State decomposition ====
x1 = x(1:2);      % q
x2 = x(3:4);      % dq
x3 = x(5:6);      % θ
x4 = x(7:8);      % dθ

a1 = m1*lc1^2 + m2*l1^2 + I1;
a2 = m2*lc2^2 + I2;
a3 = m2*l1*lc2;
a4 = (m1*lc1 + m2*l1)*g;
a5 = m2*g*lc2;
% a1 = 4.0;
% a2 = 3.5;
% a3 = 3.0;
% a4 = 39.24;
% a5 = 29.43;

% ------------------------
% State variables
% ------------------------
q1 = x(1); q2 = x(2);
dq1 = x(3); dq2 = x(4);

% ------------------------
% Mass matrix M(q)
% ------------------------
M11 = a1 + a2 + 2 * 3 * cos(q2);
M12 = a2 + a3 * cos(q2);
M21 = M12;
M22 = a2;

M0 = [M11, M12;
     M21, M22];

% ------------------------
% Coriolis/centrifugal matrix C(q, dq)
% ------------------------
C11 = -a3 * dq2 * sin(q2);
C12 = -a3 * (dq1 + dq2) * sin(q2);
C21 =  a3 * dq1 * sin(q2);
C22 = 0;

C0 = [C11, C12;
     C21, C22];

% ------------------------
% Gravity term G(q)
% ------------------------
G1 = a4 * sin(q1) + a5 * sin(q1 + q2);
G2 = a5 * sin(q1 + q2);
G0 = [G1;
     G2];

% ------------------------
c1 = diag([25, 25]);
c2 = diag([20, 20]);
c3 = diag([15, 15]);

% ==== Layer 1 ====
e1 = x1 - xd;
v1 = e1 - xi1;
alpha1 = -k1 * v1 + dxd - c1 *xi1;

dz1  = z1d;
dz1d = -2 * zeta * omega_n * z1d - omega_n^2 * (z1 - alpha1);

d_xi1 = -c1 * xi1 + xi2 + (z1 - alpha1);

% ==== Layer 2 ====
e2 = x2 - z1;
v2 = e2 - xi2;
alpha2 = K0 \ ( -k2 * v2 -c2 * xi2 + M0 * z1d - M0 * w1_hat + C0 * z1 + G0 + K0 * x1  - v1 );

dz2  = z2d;
dz2d = -2 * zeta * omega_n * z2d - omega_n^2 * (z2 - alpha2);

d_xi2 = M0 \ ( - c2 * xi2 + K0 * xi3 + K0 * (z2 - alpha2) + C0 * xi2);
v2 = e2 - xi2;

% ==== Layer 3 ====
e3 = x3 - z2;
v3 = e3 - xi3;

alpha3 = -k3 * v3 + z2d - K0 * v2 - c3 * xi3;

dz3  = z3d;
dz3d = -2 * zeta * omega_n * z3d - omega_n^2 * (z3 - alpha3);

d_xi3 = -c3 * xi3 + xi4 + (z3 - alpha3);

% ==== Layer 4 ====
e4 = x4 - z3;
v4 = e4 - xi4;
u =  -k4 * v4 - K0 * (x1 - x3) + J0 * z3d - v3 - J0 * w2_hat;
test = G0;
d_xi4 = 0;

% u = 100 * tanh(u / 100);  % smooth saturation
end

== matlab function stablechange/MATLAB Function4 ==
  data: q1 input; x output; q2 input; dq1 input; dq2 input; th1 input; th2 input; dth1 input; dth2 input
function x = pack_state(q1, q2, dq1, dq2, th1, th2, dth1, dth2)
    x = [q1; q2; dq1; dq2; th1; th2; dth1; dth2];
end
